simulink model "SF103A_MotRefMdl"  (R2013b)
settings: Solver=FixedStepDiscrete  StartTime=0.0  StopTime=2  FixedStep=.002  RelTol=1e-3
values from neighbouring files (symbols this model uses):
  ARCHGLBPRM_2MILLISEC_SEC_F32 = DataDict.Constant    [SF103A_MotRefMdl_DataDict.m]
  ARCHGLBPRM_2OVERSQRT3_ULS_F32 = DataDict.Constant    [SF103A_MotRefMdl_DataDict.m]
  ARCHGLBPRM_2PI_ULS_F32 = DataDict.Constant    [SF103A_MotRefMdl_DataDict.m]
  ARCHGLBPRM_4OVERSQRT3_ULS_F32 = DataDict.Constant    [SF103A_MotRefMdl_DataDict.m]
  ARCHGLBPRM_5PIOVER4_ULS_F32 = DataDict.Constant    [SF103A_MotRefMdl_DataDict.m]
  ARCHGLBPRM_FLOATZEROTHD_ULS_F32 = DataDict.Constant    [SF103A_MotRefMdl_DataDict.m]
  ARCHGLBPRM_HALFSQRT3_ULS_F32 = DataDict.Constant    [SF103A_MotRefMdl_DataDict.m]
  ARCHGLBPRM_PI_ULS_F32 = DataDict.Constant    [SF103A_MotRefMdl_DataDict.m]
  MotRefMdlCurrDaxBoostGain = DataDict.Calibration    [SF103A_MotRefMdl_DataDict.m]
  MotRefMdlCurrDaxQaxRefDelta = DataDict.Calibration    [SF103A_MotRefMdl_DataDict.m]
  MotRefMdlCurrItrnTolr = DataDict.Calibration    [SF103A_MotRefMdl_DataDict.m]
  MotRefMdlFbCtrlDi = DataDict.Calibration    [SF103A_MotRefMdl_DataDict.m]
  MotRefMdlIvtrDeadTiBrdgVltgSca = DataDict.Calibration    [SF103A_MotRefMdl_DataDict.m]
  MotRefMdlMinCurrItrnLim = DataDict.Calibration    [SF103A_MotRefMdl_DataDict.m]
  MotRefMdlMotCurrDaxMaxSca = DataDict.Calibration    [SF103A_MotRefMdl_DataDict.m]
  MotRefMdlMotVltgDerivtvTiCon = DataDict.Calibration    [SF103A_MotRefMdl_DataDict.m]
  MotRefMdlRefLocnItrnLim = DataDict.Calibration    [SF103A_MotRefMdl_DataDict.m]
  MotRefMdlTqItrnLim = DataDict.Calibration    [SF103A_MotRefMdl_DataDict.m]
  MotRefMdlTqItrnTolr = DataDict.Calibration    [SF103A_MotRefMdl_DataDict.m]
  MotRefMdlVltgModDynCmpEna = DataDict.Calibration    [SF103A_MotRefMdl_DataDict.m]
  MotRefMdlVltgOverRThdSca = DataDict.Calibration    [SF103A_MotRefMdl_DataDict.m]
  SysGlbPrmMotPoleCnt = DataDict.ImprtdCal    [SF103A_MotRefMdl_DataDict.m]
undefined symbols (not defined in the file or in its folder): MotQuad1
libraries: NxtrLim x19, simulink x4, LnrIntrpn x3, Fil x2, NxtrAbslt x2, FixdToFloat x2, FloatToFixd x2, NxtrMath x1
(part 1 of 7)
settings Model: Creator=lzz0tm  LastModifiedBy=RZ2YLP
settings DataIOCC: LimitDataPoints=off  SaveFormat=Structure  SignalLogging=off  DSMLogging=off
settings OptimizationCC: BlockReduction=off  InlineParams=on  ZeroExternalMemoryAtStartup=off  ZeroInternalMemoryAtStartup=off  OptimizeModelRefInitCode=on  LifeSpan=1
settings DebuggingCC: SignalInfNanChecking=error  SignalRangeChecking=warning  UnderspecifiedInitializationDetection=Simplified  SolverPrmCheckMsg=error  InheritedTsInSrcMsg=error  DiscreteInheritContinuousMsg=error  SingleTaskRateTransMsg=error  TasksWithSamePriorityMsg=error  SigSpecEnsureSampleTimeMsg=error  CheckMatrixSingularityMsg=error  IntegerOverflowMsg=error  ParameterUnderflowMsg=error  ParameterPrecisionLossMsg=error  ParameterTunabilityLossMsg=error  FixptConstUnderflowMsg=warning  FixptConstOverflowMsg=warning  VectorMatrixConversionMsg=error  SignalLabelMismatchMsg=error  UnconnectedInputMsg=error  UnconnectedOutputMsg=error  UnconnectedLineMsg=error  SFcnCompatibilityMsg=error  UniqueDataStoreMsg=warning  BusObjectLabelMismatch=error  RootOutportRequireBusObject=error  AssertControl=DisableAll  ModelReferenceIOMsg=error  ModelReferenceVersionMismatchMessage=warning  ModelReferenceIOMismatchMessage=error  ModelReferenceCSMismatchMessage=warning  ModelReferenceDataLoggingMessage=error  StateNameClashWarn=warning  StrictBusMsg=ErrorOnBusTreatedAsVector  NonBusSignalsTreatedAsBus=error  SFUnexpectedBacktrackingDiag=error  SFInvalidInputDataAccessInChartInitDiag=error  SFNoUnconditionalDefaultTransitionDiag=error  SFTransitionOutsideNaturalParentDiag=error  SFUnconditionalTransitionShadowingDiag=error  SFUndirectedBroadcastEventsDiag=error
settings ModelReferenceCC: ModelReferenceNumInstancesAllowed=Single
settings RTWCC: SystemTargetFile=autosar.tlc  GenCodeOnly=on  TemplateMakefile=ert_default_tmf  Description=AUTOSAR  GenerateReport=on  ProcessScript=autosar_make_rtw_hook  LaunchReport=on
settings CodeAppCC: GenerateComments=off  IgnoreCustomStorageClasses=off  CustomSymbolStrType=$N$R$M  CustomSymbolStrBlkIO=$N$M  SimulinkBlockComments=off
settings STFCustomTargetCC: ParMdlRefBuildCompliant=on  CompOptLevelCompliant=on  IncludeMdlTerminateFcn=off  CombineOutputUpdateFcns=on  SuppressErrorStatus=on  ERTFirstTimeCompliant=on  ERTCustomFileBanners=on  SupportNonFinite=off  SupportComplex=off  SupportContinuousTime=off  SupportNonInlinedSFcns=off  MATLABClassNameForMDSCustomization=Simulink.SoftwareTarget.ERTCustomization  AutosarCompliant=on  GRTInterface=off  SystemTargetFile=autosar.tlc
settings ERTTargetCC: CodeReplacementLibrary=ANSI_C  ConcurrentExecutionCompliant=off  IncludeMdlTerminateFcn=off  SuppressErrorStatus=on  SupportNonFinite=off  SupportComplex=off  ModelStepFunctionPrototypeControlCompliant=off  CPPClassGenCompliant=off  AutosarCompliant=on  InlinedParameterPlacement=NonHierarchical  ERTCustomFileTemplate=example_file_process.tlc  EnableUserReplacementTypes=on

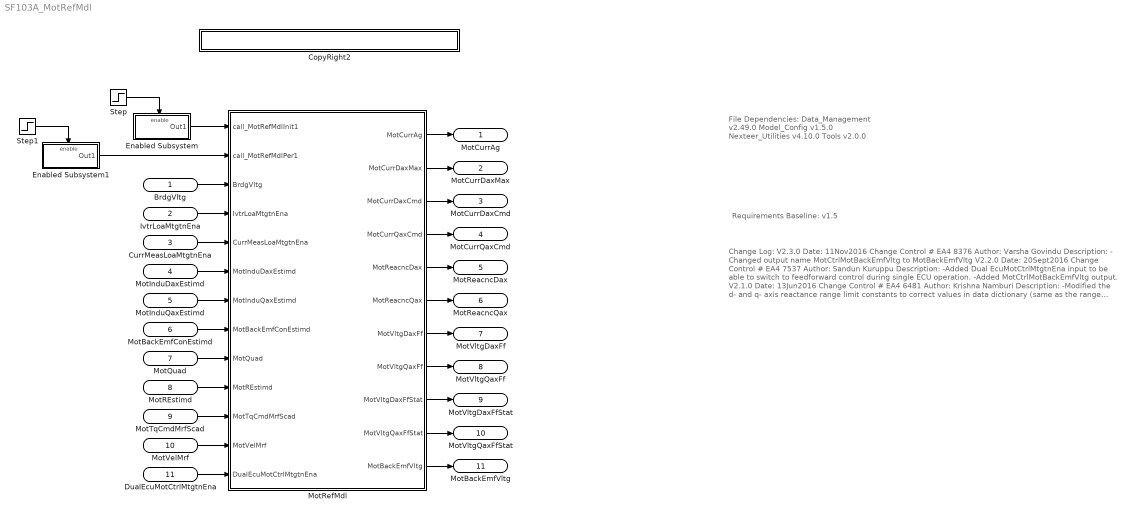
== system SF103A_MotRefMdl ==
  note: Requirements Baseline: v1.5
  note: File Dependencies:
      |
      | Data_Management v2.49.0
      | Model_Config v1.5.0
      | Nexteer_Utilities v4.10.0
      | Tools v2.0.0
  note: Change Log:
      |
      | V2.3.0
      | Date: 11Nov2016
      | Change Control # EA4 8376
      | Author: Varsha Govindu
      | Description:
      | - Changed  output name MotCtrlMotBackEmfVltg to MotBackEmfVltg
      |
      |
      | V2.2.0
      | Date: 20Sept2016
      | Change Control # EA4 7537
      | Author: Sandun Kuruppu
      | Description:
      | -Added Dual EcuMotCtrlMtgtnEna input to be able to switch to feedforward control during single
      | ECU operation.
      | -Added MotCtrlMotBackEmfVltg output.
      |
      | V2.1.0
      | Date: 13Jun2016
      | Change Control # EA4 6481
      | Author: Krishna Namburi
      | Description:
      | -Modified the d- and q- axis reactance range limit constants to correct values in data dictionary
      | (same as the range specified for the corresponding output signals).
      | -Corrected theDOORS requirement links for the output signals
      |
      | V2.0.0
      | Date: 13Jun2016
      | Change Control # EA46068
      | Author: Krishna Namburi
      | Description:
      | Added Saturation blocks to the feedforward voltage outputs.
      | Added two ouputs MotVltgDaxFfStat and MotVltgQaxFfStat
      |
      | V1.3.0
      | Date: 25Apr2016
      | Change Control: EA4#5437, EA4#5363, EA4#5505
      | DRW: Sudeep Shankar
      | Description:
      |
      | EA4#5437:
      | - Removed saturation block on the outputs MotVltgDaxFf and MotVltgQaxFf.
      | - Removed the constant  MOTVLTGLOLIM_VOLT_F32 from data dictionary as
      | it is no longer used.
      | - Changed the name of constant MOTVLTGHILIM_VOLT_F32 to
      | BRDGVLTGHILIM_VOLT_F32 in model and DD.
      | - Added saturation block on the inputs MotVelMrf and MotTqCmdMrfScad
      | - Added Motor velocity high and low limit constants and Motor Torque command
      | high and low limit constants in data dictionary.
      |
      | EA4#5363:
      | - Changed the name of the input signal 'MotCurrLoaMtgtnEna' to
      | 'CurrMeasLoaMtgtnEna' both in design and datadictionary
      |
      | EA4#5505:
      | - Added display variables for MotVltgDaxFfStat and MotVltgQaxFfStat
      |
      | V1.2.0
      | Date: 14Mar2016
      | Change Control: EA4#4665
      | DRW: Muragesh Asundi(KPIT)
      | Description:
      | Changed signal name from "MotCtrlMotCurrLoaMtgtnEna" to
      |  "MotCurrLoaMtgtnEna".
      |
      | V1.1.0
      | Date: 12Feb2016
      | Change Control: EA4#6578
      | DRW: Shailesh/Hemlata kamble/Muragesh(KPIT)
      | Description:
      | 1. Changed the inputs for calculation of "MotCurrDaxMax".
      | Used "MotInduDaxEstimd" instead of "MotInduQaxEstimd" as per EA4#2360
      | 2.Replaced "limiter block" with "if-else" logic as mentioned in EA4#2665
      | 3. Names of following have corrected as per AUTOSAR naming convention
      |
      | MotRefMdlCurrIterTol -> MotRefMdlCurrItrnTolr
      | MotRefMdlMinCurrIterLim -> MotRefMdlMinCurrItrnLim
      | MotRefMdlQ13VltgSdlX -> MotRefMdlQuad13VltgSdlX
      | MotRefMdlQ13VltgSdlY -> MotRefMdlQuad13VltgSdlY
      | MotRefMdlQ24VltgSdlX -> MotRefMdlQuad24VltgSdlX
      | MotRefMdlQ24VltgSdlY -> MotRefMdlQuad24VltgSdlY
      | MotRefMdlRefLocnIterLim -> MotRefMdlRefLocnItrnLim
      | MotRefMdlTqIterLim -> MotRefMdlTqItrnLim
      | MotRefMdlTqIterTol -> MotRefMdlTqItrnTolr
      | MotRefMdlVltgOvrRThdSca - MotRefMdlVltgOverRThdSca
      | dMotRefMdlPkTqNrItrn -> dMotRefMdlPeakTqNrItrn
      |
      | V1.0.0
      | Date: 19june2015
      | Change Control: EA4#285
      | DRW: Kevin Derry
      | Description:
      | - Initial Release
  BrdgVltg : Inport  RequirementInfo={} %GIDa_002e74ba_4d90_44d4_90c6_7a7ed3b84fe7
  IvtrLoaMtgtnEna : Inport  RequirementInfo={} %GIDa_a4fd61a5_cdd6_4e13_bb24_ad86140a0e25  Port=2
  CurrMeasLoaMtgtnEna : Inport  RequirementInfo={} %GIDa_c2a4c68b_2d87_4ecb_ac32_cc9aba368d56  Port=3
  MotInduDaxEstimd : Inport  RequirementInfo={} %GIDa_fe459d42_11f7_4520_8391_798b83d6a516  Port=4
  MotInduQaxEstimd : Inport  RequirementInfo={} %GIDa_0f6b35e5_2a2f_4a67_b96e_911dafdf4a7c  Port=5
  MotBackEmfConEstimd : Inport  RequirementInfo={} %GIDa_5b757b48_21e1_4bdd_bbe8_b25eaabed28d  Port=6
  MotQuad : Inport  RequirementInfo={} %GIDa_e10e4028_772a_461b_a96b_8e88bd788124  Port=7
  MotREstimd : Inport  RequirementInfo={} %GIDa_daff92ee_9fcb_4c1d_949c_c1b84c0d8058  Port=8
  MotTqCmdMrfScad : Inport  RequirementInfo={} %GIDa_5a505ccf_fd01_460a_b553_b9760a103946  Port=9
  MotVelMrf : Inport  RequirementInfo={} %GIDa_3a206742_0817_4b89_aaee_a915b460cff8  Port=10
  DualEcuMotCtrlMtgtnEna : Inport  RequirementInfo={} %GIDa_c709b502_2fd2_4013_acca_47a6e0722eaa  Port=11
  CopyRight2 : Subsystem  Description=|  mask(Copyright Information){none=on}
      | Copyright info block.                                               
      |                                                                     
      | Place copyright information at the top of every subsystem in design.
      mask prompts: none "No parameters"
      mask help: Place copyright information at the top of every subsystem in design.
      mask Display:
      | NxtrConf = 'Nexteer Confidential';
      | 
      | sys = bdroot; %handle for the current model ("system")
      | first = get_param(sys,'Created');
      | first = first(end-3:end);  %year is last four digits
      | 
      | last = get_param(sys,'LastModifiedDate');
      | if isempty(last)
      |     last = datestr(now,'yyyy');
      | else
      |     last = last(end-3:end);
      | end
      | 
      | if strcmp(first,last)
      |     fprintf('%s -- Copyright %s Nexteer',NxtrConf,first)
      | else
      |     fprintf('%s -- %s%s- %s Nexteer',NxtrConf,char(169),first,last)
      | end
  Enabled Subsystem : Subsystem  RequirementInfo={} %GIDa_5bd5b926_dcf2_442a_84c3_2b04d7299c9b  TreatAsAtomicUnit=on
  Enabled Subsystem1 : Subsystem  RequirementInfo={} %GIDa_aef5c3eb_1d89_4c7b_a89d_5c18a3b0f7b1  TreatAsAtomicUnit=on
  MotRefMdl : Subsystem  RequirementInfo={} %GIDa_b898030d_570f_4edd_8902_3dde318359c9
      settings: AttributesFormatString=%<Tag>
  Step : Step  RequirementInfo={} %GIDa_8c81d09d_84eb_4be8_baaa_75d0e6280a38  Time=.00001  Before=1  After=0  SampleTime=0.002
  Step1 : Step  RequirementInfo={} %GIDa_d7228de7_f622_4d51_9092_7c3999a0281d  Time=.00001  SampleTime=0.002
  MotCurrAg : Outport  RequirementInfo={} %GIDa_93cad014_54f9_4783_990f_6d2e5aad039b
  MotCurrDaxMax : Outport  RequirementInfo={} %GIDa_4136d505_73be_4586_8175_3cca54354780  Port=2
  MotCurrDaxCmd : Outport  RequirementInfo={} %GIDa_75f52d22_fe2b_494b_ac4f_7f4b1e1c25cf  Port=3
  MotCurrQaxCmd : Outport  RequirementInfo={} %GIDa_eb935c6c_ac14_4f59_8619_b2ab2e4003c8  Port=4
  MotReacncDax : Outport  RequirementInfo={} %GIDa_5d917e0d_38b8_4778_841b_e252e5a24515  Port=5
  MotReacncQax : Outport  RequirementInfo={} %GIDa_4b30cc88_72f0_4383_99ae_c006978f770d  Port=6
  MotVltgDaxFf : Outport  RequirementInfo={} %GIDa_44799714_324f_4cb8_bf73_cca9c6cf36e6  Port=7
  MotVltgQaxFf : Outport  RequirementInfo={} %GIDa_4412ce0c_324b_49e2_9e94_75936e15aac2  Port=8
  MotVltgDaxFfStat : Outport  RequirementInfo={} %GIDa_9d33dac4_1325_4267_bc65_d009f3dffb61  Port=9
  MotVltgQaxFfStat : Outport  RequirementInfo={} %GIDa_1d00fc51_e529_4e10_8bf6_e979105e5d3e  Port=10
  MotBackEmfVltg : Outport  RequirementInfo={} %GIDa_d7c5f473_23d1_4699_ab39_3d8c13b39e2e  Port=11
  wires:
  Enabled Subsystem1/1(Out1) -> MotRefMdl/2(call_MotRefMdlPer1)
  Enabled Subsystem/1(Out1) -> MotRefMdl/1(call_MotRefMdlInit1)
  Step/1 -> Enabled Subsystem/Enable
  MotRefMdl/6(MotReacncQax) -> MotReacncQax/1
  MotRefMdl/8(MotVltgQaxFf) -> MotVltgQaxFf/1
  MotRefMdl/7(MotVltgDaxFf) -> MotVltgDaxFf/1
  MotRefMdl/2(MotCurrDaxMax) -> MotCurrDaxMax/1
  MotRefMdl/4(MotCurrQaxCmd) -> MotCurrQaxCmd/1
  MotRefMdl/5(MotReacncDax) -> MotReacncDax/1
  MotRefMdl/3(MotCurrDaxCmd) -> MotCurrDaxCmd/1
  MotRefMdl/1(MotCurrAg) -> MotCurrAg/1
  CurrMeasLoaMtgtnEna/1 -> MotRefMdl/5(CurrMeasLoaMtgtnEna)
  MotInduQaxEstimd/1 -> MotRefMdl/7(MotInduQaxEstimd)
  IvtrLoaMtgtnEna/1 -> MotRefMdl/4(IvtrLoaMtgtnEna)
  MotInduDaxEstimd/1 -> MotRefMdl/6(MotInduDaxEstimd)
  MotBackEmfConEstimd/1 -> MotRefMdl/8(MotBackEmfConEstimd)
  BrdgVltg/1 -> MotRefMdl/3(BrdgVltg)
  MotQuad/1 -> MotRefMdl/9(MotQuad)
  MotREstimd/1 -> MotRefMdl/10(MotREstimd)
  MotVelMrf/1 -> MotRefMdl/12(MotVelMrf)
  MotTqCmdMrfScad/1 -> MotRefMdl/11(MotTqCmdMrfScad)
  MotRefMdl/10(MotVltgQaxFfStat) -> MotVltgQaxFfStat/1
  MotRefMdl/9(MotVltgDaxFfStat) -> MotVltgDaxFfStat/1
  MotRefMdl/11(MotBackEmfVltg) -> MotBackEmfVltg/1
  DualEcuMotCtrlMtgtnEna/1 -> MotRefMdl/13(DualEcuMotCtrlMtgtnEna)
  Step1/1 -> Enabled Subsystem1/Enable

== system SF103A_MotRefMdl/CopyRight2 ==

== system SF103A_MotRefMdl/Enabled Subsystem ==
  Enable : EnablePort
  Function-Call Generator : simulink/Ports & Subsystems/Function-Call Generator  sample_time=.002  numberOfIterations=1
  Out1 : Outport
  wires:
  Function-Call Generator/1 -> Out1/1

== system SF103A_MotRefMdl/Enabled Subsystem1 ==
  Enable : EnablePort
  Function-Call Generator : simulink/Ports & Subsystems/Function-Call Generator  sample_time=.002  numberOfIterations=1
  Out1 : Outport
  wires:
  Function-Call Generator/1 -> Out1/1

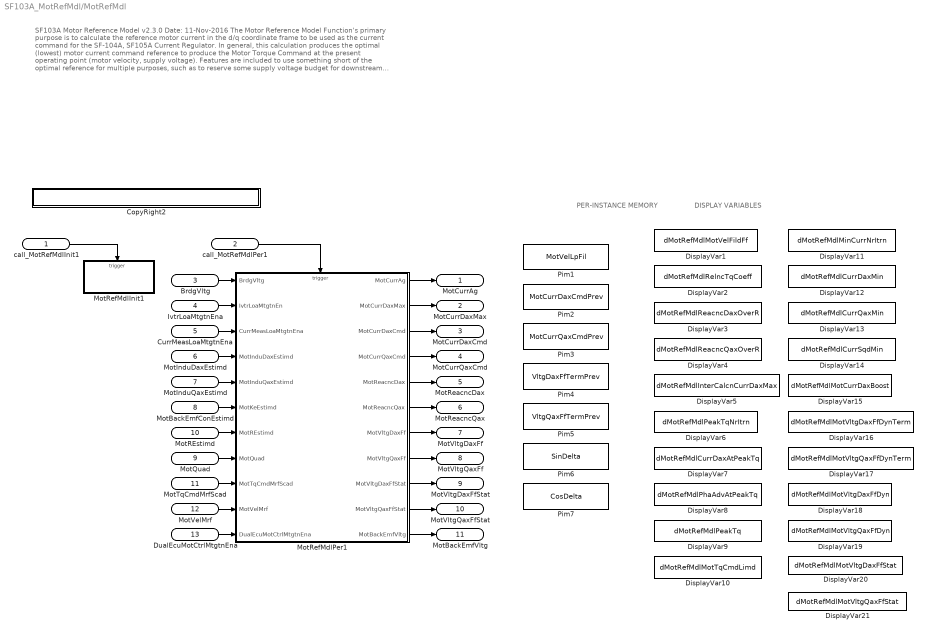
== system SF103A_MotRefMdl/MotRefMdl ==
  note: DISPLAY VARIABLES
  note: PER-INSTANCE
      | MEMORY
  note: SF103A  Motor Reference Model
      | v2.3.0      Date: 11-Nov-2016
      |
      | The Motor Reference Model Function's primary purpose is to calculate the reference motor current in the d/q coordinate frame to
      | be used as the current command for the SF-104A, SF105A Current Regulator.  In general, this calculation produces the optimal
      | (lowest) motor current command reference to produce the Motor Torque Command at the present operating point (motor velocity,
      |  supply voltage).  Features are included to use something short of the optimal reference for multiple purposes, such as to reserve
      |  some supply voltage budget for downstream current regulator operation, or for cogging/ripple cancellation, or to smooth the transition
      |  of low values of Id to high values of Id as the motor operating conditions change.  Supplementary functions include the calculation of a
      | Feedforward Reference Voltage for use in the SF-105A Current Regulator, whose form changes depending on the state of the signa
      | l LoA State (this allows operation in Voltage Mode Control in certain fail operational states).  Another supplementary function computes the
      |  Motor Reference Current angle (Alpha) for use in the Current Measurement function.
  call_MotRefMdlInit1 : Inport
  call_MotRefMdlPer1 : Inport  Port=2
  BrdgVltg : Inport  RequirementInfo={'linktype_rmi_doors' '0000bb42 (/E-STEER Core/SubSystem Specifications/Application Functions/SF99/SF103A Motor Reference Model)' '#SF103A_42' 'true' 'REQ:SF103A_42' '' } %GIDa_d3b1f893_8188_46d5_b395_9d7b6c4fbcc4  Port=3
  IvtrLoaMtgtnEna : Inport  RequirementInfo={'linktype_rmi_doors' '0000bb42 (/E-STEER Core/SubSystem Specifications/Application Functions/SF99/SF103A Motor Reference Model)' '#SF103A_183' 'true' 'REQ:SF103A_183' '' } %GIDa_c71961af_9957_4c72_9ff9_40a82d1c1450  Port=4
  CurrMeasLoaMtgtnEna : Inport  RequirementInfo={'linktype_rmi_doors' '0000bb42 (/E-STEER Core/SubSystem Specifications/Application Functions/SF99/SF103A Motor Reference Model)' '#SF103A_43' 'true' 'REQ:SF103A_43' '' } %GIDa_24854601_cc59_47b1_bc2c_d32f45ce8169  Port=5
  MotInduDaxEstimd : Inport  RequirementInfo={'linktype_rmi_doors' '0000bb42 (/E-STEER Core/SubSystem Specifications/Application Functions/SF99/SF103A Motor Reference Model)' '#SF103A_39' 'true' 'REQ:SF103A_39' '' } %GIDa_d84c7e48_30a1_4e89_aeaa_9b2784ab142a  Port=6
  MotInduQaxEstimd : Inport  RequirementInfo={'linktype_rmi_doors' '0000bb42 (/E-STEER Core/SubSystem Specifications/Application Functions/SF99/SF103A Motor Reference Model)' '#SF103A_40' 'true' 'REQ:SF103A_40' '' } %GIDa_2edb5c24_fcdf_496b_ab32_7ad89ca27fdb  Port=7
  MotBackEmfConEstimd : Inport  RequirementInfo={'linktype_rmi_doors' '0000bb42 (/E-STEER Core/SubSystem Specifications/Application Functions/SF99/SF103A Motor Reference Model)' '#SF103A_37' 'true' 'REQ:SF103A_37' '' } %GIDa_5a4a70dc_38a8_4966_aa75_58c98909303e  Port=8
  MotQuad : Inport  RequirementInfo={'linktype_rmi_doors' '0000bb42 (/E-STEER Core/SubSystem Specifications/Application Functions/SF99/SF103A Motor Reference Model)' '#SF103A_41' 'true' 'REQ:SF103A_41' '' } %GIDa_acb8662c_f7ec_4e47_adb3_a0fa4bbfd4b9  Port=9
  MotREstimd : Inport  RequirementInfo={'linktype_rmi_doors' '0000bb42 (/E-STEER Core/SubSystem Specifications/Application Functions/SF99/SF103A Motor Reference Model)' '#SF103A_38' 'true' 'REQ:SF103A_38' '' } %GIDa_d7c155ac_593d_4c0d_b2cd_a76dbcfddff9  Port=10
  MotTqCmdMrfScad : Inport  RequirementInfo={'linktype_rmi_doors' '0000bb42 (/E-STEER Core/SubSystem Specifications/Application Functions/SF99/SF103A Motor Reference Model)' '#SF103A_27' 'true' 'REQ:SF103A_27' '' } %GIDa_3d3c202a_f654_45d5_8a5b_acbb1c7e6aa0  Port=11
  MotVelMrf : Inport  RequirementInfo={'linktype_rmi_doors' '0000bb42 (/E-STEER Core/SubSystem Specifications/Application Functions/SF99/SF103A Motor Reference Model)' '#SF103A_36' 'true' 'REQ:SF103A_36' '' } %GIDa_7d8dfaf1_29d4_42ed_9984_abcaa0131fe4  Port=12
  DualEcuMotCtrlMtgtnEna : Inport  RequirementInfo={'linktype_rmi_doors' '0000bb42 (/E-STEER Core/SubSystem Specifications/Application Functions/SF99/SF103A Motor Reference Model)' '#SF103A_36' 'true' 'REQ:SF103A_36' '' } %GIDa_62cd6ed4_e69a_42ee_9441_e0d528756875  Port=13
  CopyRight2 : Subsystem  Description=|  mask(Copyright Information){none=on}
      | Copyright info block.                                               
      |                                                                     
      | Place copyright information at the top of every subsystem in design.
      mask prompts: none "No parameters"
      mask help: Place copyright information at the top of every subsystem in design.
      mask Display:
      | NxtrConf = 'Nexteer Confidential';
      | 
      | sys = bdroot; %handle for the current model ("system")
      | first = get_param(sys,'Created');
      | first = first(end-3:end);  %year is last four digits
      | 
      | last = get_param(sys,'LastModifiedDate');
      | if isempty(last)
      |     last = datestr(now,'yyyy');
      | else
      |     last = last(end-3:end);
      | end
      | 
      | if strcmp(first,last)
      |     fprintf('%s -- Copyright %s Nexteer',NxtrConf,first)
      | else
      |     fprintf('%s -- %s%s- %s Nexteer',NxtrConf,char(169),first,last)
      | end
  DisplayVar1 : DataStoreMemory  DataStoreName=dMotRefMdlMotVelFildFf  ReadBeforeWriteMsg=warning  WriteAfterWriteMsg=warning  WriteAfterReadMsg=warning  StateMustResolveToSignalObject=on
  DisplayVar10 : DataStoreMemory  DataStoreName=dMotRefMdlMotTqCmdLimd  ReadBeforeWriteMsg=warning  WriteAfterWriteMsg=warning  WriteAfterReadMsg=warning  StateMustResolveToSignalObject=on
  DisplayVar11 : DataStoreMemory  DataStoreName=dMotRefMdlMinCurrNrItrn  ReadBeforeWriteMsg=warning  WriteAfterWriteMsg=warning  WriteAfterReadMsg=warning  StateMustResolveToSignalObject=on
  DisplayVar12 : DataStoreMemory  DataStoreName=dMotRefMdlCurrDaxMin  ReadBeforeWriteMsg=warning  WriteAfterWriteMsg=warning  WriteAfterReadMsg=warning  StateMustResolveToSignalObject=on
  DisplayVar13 : DataStoreMemory  DataStoreName=dMotRefMdlCurrQaxMin  ReadBeforeWriteMsg=warning  WriteAfterWriteMsg=warning  WriteAfterReadMsg=warning  StateMustResolveToSignalObject=on
  DisplayVar14 : DataStoreMemory  DataStoreName=dMotRefMdlCurrSqdMin  ReadBeforeWriteMsg=warning  WriteAfterWriteMsg=warning  WriteAfterReadMsg=warning  StateMustResolveToSignalObject=on
  DisplayVar15 : DataStoreMemory  DataStoreName=dMotRefMdlMotCurrDaxBoost  ReadBeforeWriteMsg=warning  WriteAfterWriteMsg=warning  WriteAfterReadMsg=warning  StateMustResolveToSignalObject=on
  DisplayVar16 : DataStoreMemory  DataStoreName=dMotRefMdlMotVltgDaxFfDynTerm  ReadBeforeWriteMsg=warning  WriteAfterWriteMsg=warning  WriteAfterReadMsg=warning  StateMustResolveToSignalObject=on
  DisplayVar17 : DataStoreMemory  DataStoreName=dMotRefMdlMotVltgQaxFfDynTerm  ReadBeforeWriteMsg=warning  WriteAfterWriteMsg=warning  WriteAfterReadMsg=warning  StateMustResolveToSignalObject=on
  DisplayVar18 : DataStoreMemory  DataStoreName=dMotRefMdlMotVltgDaxFfDyn  ReadBeforeWriteMsg=warning  WriteAfterWriteMsg=warning  WriteAfterReadMsg=warning  StateMustResolveToSignalObject=on
  DisplayVar19 : DataStoreMemory  DataStoreName=dMotRefMdlMotVltgQaxFfDyn  ReadBeforeWriteMsg=warning  WriteAfterWriteMsg=warning  WriteAfterReadMsg=warning  StateMustResolveToSignalObject=on
  DisplayVar2 : DataStoreMemory  DataStoreName=dMotRefMdlRelncTqCoeff  ReadBeforeWriteMsg=warning  WriteAfterWriteMsg=warning  WriteAfterReadMsg=warning  StateMustResolveToSignalObject=on
  DisplayVar20 : DataStoreMemory  DataStoreName=dMotRefMdlMotVltgDaxFfStat  ReadBeforeWriteMsg=warning  WriteAfterWriteMsg=warning  WriteAfterReadMsg=warning  StateMustResolveToSignalObject=on
  DisplayVar21 : DataStoreMemory  DataStoreName=dMotRefMdlMotVltgQaxFfStat  ReadBeforeWriteMsg=warning  WriteAfterWriteMsg=warning  WriteAfterReadMsg=warning  StateMustResolveToSignalObject=on
  DisplayVar3 : DataStoreMemory  DataStoreName=dMotRefMdlReacncDaxOverR  ReadBeforeWriteMsg=warning  WriteAfterWriteMsg=warning  WriteAfterReadMsg=warning  StateMustResolveToSignalObject=on
  DisplayVar4 : DataStoreMemory  DataStoreName=dMotRefMdlReacncQaxOverR  ReadBeforeWriteMsg=warning  WriteAfterWriteMsg=warning  WriteAfterReadMsg=warning  StateMustResolveToSignalObject=on
  DisplayVar5 : DataStoreMemory  DataStoreName=dMotRefMdlInterCalcnCurrDaxMax  ReadBeforeWriteMsg=warning  WriteAfterWriteMsg=warning  WriteAfterReadMsg=warning  StateMustResolveToSignalObject=on
  DisplayVar6 : DataStoreMemory  DataStoreName=dMotRefMdlPeakTqNrItrn  ReadBeforeWriteMsg=warning  WriteAfterWriteMsg=warning  WriteAfterReadMsg=warning  StateMustResolveToSignalObject=on
  DisplayVar7 : DataStoreMemory  DataStoreName=dMotRefMdlCurrDaxAtPeakTq  ReadBeforeWriteMsg=warning  WriteAfterWriteMsg=warning  WriteAfterReadMsg=warning  StateMustResolveToSignalObject=on
  DisplayVar8 : DataStoreMemory  DataStoreName=dMotRefMdlPhaAdvAtPeakTq  ReadBeforeWriteMsg=warning  WriteAfterWriteMsg=warning  WriteAfterReadMsg=warning  StateMustResolveToSignalObject=on
  DisplayVar9 : DataStoreMemory  DataStoreName=dMotRefMdlPeakTq  ReadBeforeWriteMsg=warning  WriteAfterWriteMsg=warning  WriteAfterReadMsg=warning  StateMustResolveToSignalObject=on
  MotRefMdlInit1 : Subsystem  TreatAsAtomicUnit=on
  MotRefMdlPer1 : Subsystem  TreatAsAtomicUnit=on
  Pim1 : DataStoreMemory  DataStoreName=MotVelLpFil  InitialValue=struct('FilSt',single(0),'FilGain',single(0))  OutDataTypeStr=Bus: FilLpRec1  StateMustResolveToSignalObject=on
  Pim2 : DataStoreMemory  DataStoreName=MotCurrDaxCmdPrev  WriteAfterWriteMsg=warning  StateMustResolveToSignalObject=on
  Pim3 : DataStoreMemory  DataStoreName=MotCurrQaxCmdPrev  WriteAfterWriteMsg=warning  StateMustResolveToSignalObject=on
  Pim4 : DataStoreMemory  DataStoreName=VltgDaxFfTermPrev  WriteAfterWriteMsg=warning  StateMustResolveToSignalObject=on
  Pim5 : DataStoreMemory  DataStoreName=VltgQaxFfTermPrev  WriteAfterWriteMsg=warning  StateMustResolveToSignalObject=on
  Pim6 : DataStoreMemory  DataStoreName=SinDelta  WriteAfterWriteMsg=warning  InitialValue=[0 0 0 0 0 0 0 0]  StateMustResolveToSignalObject=on
  Pim7 : DataStoreMemory  DataStoreName=CosDelta  WriteAfterWriteMsg=warning  InitialValue=[0 0 0 0 0 0 0 0]  StateMustResolveToSignalObject=on
  MotCurrAg : Outport  RequirementInfo={'linktype_rmi_doors' '0000bb42 (/E-STEER Core/SubSystem Specifications/Application Functions/SF99/SF103A Motor Reference Model)' '#SF103A_28' 'true' 'REQ:SF103A_28' '' } %GIDa_834cbc2e_f18c_4f09_adae_97704fe7531a
  MotCurrDaxMax : Outport  RequirementInfo={'linktype_rmi_doors' '0000bb42 (/E-STEER Core/SubSystem Specifications/Application Functions/SF99/SF103A Motor Reference Model)' '#SF103A_50' 'true' 'REQ:SF103A_50' '' } %GIDa_0574a43c_0095_465e_bbc3_0acf9fa9b1b8  Port=2
  MotCurrDaxCmd : Outport  RequirementInfo={'linktype_rmi_doors' '0000bb42 (/E-STEER Core/SubSystem Specifications/Application Functions/SF99/SF103A Motor Reference Model)' '#SF103A_45' 'true' 'REQ:SF103A_45' '' } %GIDa_fb157a0c_9e0a_4510_ba81_91b763a1b3b4  Port=3
  MotCurrQaxCmd : Outport  RequirementInfo={'linktype_rmi_doors' '0000bb42 (/E-STEER Core/SubSystem Specifications/Application Functions/SF99/SF103A Motor Reference Model)' '#SF103A_44' 'true' 'REQ:SF103A_44' '' } %GIDa_ec3cc1cf_2433_46bf_a532_04cbfbe0ffa2  Port=4
  MotReacncDax : Outport  RequirementInfo={'linktype_rmi_doors' '0000bb42 (/E-STEER Core/SubSystem Specifications/Application Functions/SF99/SF103A Motor Reference Model)' '#SF103A_49' 'true' 'REQ:SF103A_49' '' } %GIDa_97e983dd_3b16_40dc_8e10_e6499980e643  Port=5
  MotReacncQax : Outport  RequirementInfo={'linktype_rmi_doors' '0000bb42 (/E-STEER Core/SubSystem Specifications/Application Functions/SF99/SF103A Motor Reference Model)' '#SF103A_48' 'true' 'REQ:SF103A_48' '' } %GIDa_ad59918e_bb5f_4124_9238_114ac982f978  Port=6
  MotVltgDaxFf : Outport  RequirementInfo={'linktype_rmi_doors' '0000bb42 (/E-STEER Core/SubSystem Specifications/Application Functions/SF99/SF103A Motor Reference Model)' '#SF103A_47' 'true' 'REQ:SF103A_47' '' } %GIDa_a89b73f7_0999_4306_87c4_354c6cee061c  Port=7
  MotVltgQaxFf : Outport  RequirementInfo={'linktype_rmi_doors' '0000bb42 (/E-STEER Core/SubSystem Specifications/Application Functions/SF99/SF103A Motor Reference Model)' '#SF103A_46' 'true' 'REQ:SF103A_46' '' } %GIDa_3b2f5587_35c7_4629_a038_bbfce1200d31  Port=8
  MotVltgDaxFfStat : Outport  RequirementInfo={'linktype_rmi_doors' '0000bb42 (/E-STEER Core/SubSystem Specifications/Application Functions/SF99/SF103A Motor Reference Model)' '#SF103A_185' 'true' 'REQ:SF103A_185' '' } %GIDa_966cb850_afba_44e3_801f_09c3cd3e5e21  Port=9
  MotVltgQaxFfStat : Outport  RequirementInfo={'linktype_rmi_doors' '0000bb42 (/E-STEER Core/SubSystem Specifications/Application Functions/SF99/SF103A Motor Reference Model)' '#SF103A_184' 'true' 'REQ:SF103A_184' '' } %GIDa_3c4d5d68_c8f7_4475_b626_248aa50b2e24  Port=10
  MotBackEmfVltg : Outport  RequirementInfo={'linktype_rmi_doors' '0000bb42 (/E-STEER Core/SubSystem Specifications/Application Functions/SF99/SF103A Motor Reference Model)' '#SF103A_187' 'true' 'REQ:SF103A_187' '' } %GIDa_de4675c2_9a6c_40d6_a388_66e44b7ee260  Port=11
  wires:
  call_MotRefMdlInit1/1 -> MotRefMdlInit1/Trigger
  call_MotRefMdlPer1/1 -> MotRefMdlPer1/Trigger
  MotInduDaxEstimd/1 -> MotRefMdlPer1/4(MotInduDaxEstimd)
  MotTqCmdMrfScad/1 -> MotRefMdlPer1/9(MotTqCmdMrfScad)
  MotInduQaxEstimd/1 -> MotRefMdlPer1/5(MotInduQaxEstimd)
  MotVelMrf/1 -> MotRefMdlPer1/10(MotVelMrf)
  MotQuad/1 -> MotRefMdlPer1/8(MotQuad)
  IvtrLoaMtgtnEna/1 -> MotRefMdlPer1/2(IvtrLoaMtgtnEn)
  CurrMeasLoaMtgtnEna/1 -> MotRefMdlPer1/3(CurrMeasLoaMtgtnEna)
  BrdgVltg/1 -> MotRefMdlPer1/1(BrdgVltg)
  MotBackEmfConEstimd/1 -> MotRefMdlPer1/6(MotKeEstimd)
  MotREstimd/1 -> MotRefMdlPer1/7(MotREstimd)
  MotRefMdlPer1/1(MotCurrAg) -> MotCurrAg/1
  MotRefMdlPer1/7(MotVltgDaxFf) -> MotVltgDaxFf/1
  MotRefMdlPer1/2(MotCurrDaxMax) -> MotCurrDaxMax/1
  MotRefMdlPer1/6(MotReacncQax) -> MotReacncQax/1
  MotRefMdlPer1/4(MotCurrQaxCmd) -> MotCurrQaxCmd/1
  MotRefMdlPer1/3(MotCurrDaxCmd) -> MotCurrDaxCmd/1
  MotRefMdlPer1/5(MotReacncDax) -> MotReacncDax/1
  MotRefMdlPer1/8(MotVltgQaxFf) -> MotVltgQaxFf/1
  MotRefMdlPer1/10(MotVltgQaxFfStat) -> MotVltgQaxFfStat/1
  MotRefMdlPer1/9(MotVltgDaxFfStat) -> MotVltgDaxFfStat/1
  MotRefMdlPer1/11(MotBackEmfVltg) -> MotBackEmfVltg/1
  DualEcuMotCtrlMtgtnEna/1 -> MotRefMdlPer1/11(DualEcuMotCtrlMtgtnEna)

== system SF103A_MotRefMdl/MotRefMdl/CopyRight2 ==

== system SF103A_MotRefMdl/MotRefMdl/MotRefMdlInit1 ==
  note: An array of phase advance interpolation points
  function : TriggerPort  TriggerType=function-call
  Constant2 : Constant  RequirementInfo={'linktype_rmi_doors' '0000bb42 (/E-STEER Core/SubSystem Specifications/Application Functions/SF99/SF103A Motor Reference Model)' '#SF103A_92' 'true' 'REQ:SF103A_92' '' } %GIDa_da78c45d_0dc3_4ce5_ba56_4e557b79ff02  Value=MotRefMdlCurrDaxQaxRefDelta
  CopyRight2 : Subsystem  Description=|  mask(Copyright Information){none=on}
      | Copyright info block.                                               
      |                                                                     
      | Place copyright information at the top of every subsystem in design.
      mask prompts: none "No parameters"
      mask help: Place copyright information at the top of every subsystem in design.
      mask Display:
      | NxtrConf = 'Nexteer Confidential';
      | 
      | sys = bdroot; %handle for the current model ("system")
      | first = get_param(sys,'Created');
      | first = first(end-3:end);  %year is last four digits
      | 
      | last = get_param(sys,'LastModifiedDate');
      | if isempty(last)
      |     last = datestr(now,'yyyy');
      | else
      |     last = last(end-3:end);
      | end
      | 
      | if strcmp(first,last)
      |     fprintf('%s -- Copyright %s Nexteer',NxtrConf,first)
      | else
      |     fprintf('%s -- %s%s- %s Nexteer',NxtrConf,char(169),first,last)
      | end
  CosDelta : DataStoreWrite  DataStoreName=CosDelta
  FilLpInit : Fil/FilLpInit  RequirementInfo={'linktype_rmi_doors' '0000bb42 (/E-STEER Core/SubSystem Specifications/Application Functions/SF99/SF103A Motor Reference Model)' '#SF103A_132' 'true' 'REQ:SF103A_132' '' } %GIDa_a8b99e42_23aa_467e_aeec_80c45b4357e7  Ic=0  Ts=ARCHGLBPRM_2MILLISEC_SEC_F32  Freq=MotRefMdlMotVelLpFilFrq  StVar=MotVelLpFil
  SinDelta : DataStoreWrite  DataStoreName=SinDelta
  Trigonometric Function : Trigonometry  RequirementInfo={'linktype_rmi_doors' '0000bb42 (/E-STEER Core/SubSystem Specifications/Application Functions/SF99/SF103A Motor Reference Model)' '#SF103A_92' 'true' 'REQ:SF103A_92' '' } %GIDa_9d61e243_4e46_4d4f_89b1_b878dd7a23ad
  Trigonometric Function1 : Trigonometry  RequirementInfo={'linktype_rmi_doors' '0000bb42 (/E-STEER Core/SubSystem Specifications/Application Functions/SF99/SF103A Motor Reference Model)' '#SF103A_92' 'true' 'REQ:SF103A_92' '' } %GIDa_8ef282f1_90e0_42b9_ae6e_708183d3f92b  Operator=cos
  wires:
  Trigonometric Function1/1 -> CosDelta/1
  Trigonometric Function/1 -> SinDelta/1
  Constant2/1 -> Trigonometric Function1/1, Trigonometric Function/1

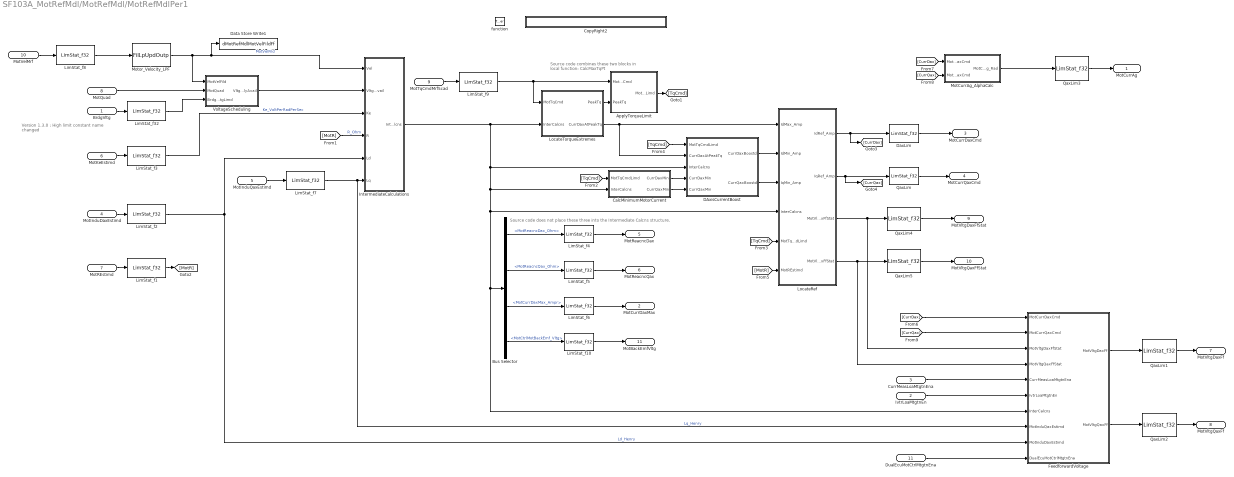
== system SF103A_MotRefMdl/MotRefMdl/MotRefMdlPer1 ==
  note: Version 1.3.0 : High limit constant name
      | changed
  note: Source code combines these two blocks
      | in local function: CalcMaxTqPt
  note: Source code does not place these three into the Intermediate Calcns structure.
  BrdgVltg : Inport
  IvtrLoaMtgtnEn : Inport  Port=2
  CurrMeasLoaMtgtnEna : Inport  Port=3
  MotInduDaxEstimd : Inport  Port=4
  MotInduQaxEstimd : Inport  Port=5
  MotKeEstimd : Inport  Port=6
  MotREstimd : Inport  Port=7
  MotQuad : Inport  Port=8
  MotTqCmdMrfScad : Inport  Port=9
  MotVelMrf : Inport  Port=10
  DualEcuMotCtrlMtgtnEna : Inport  RequirementInfo={'linktype_rmi_doors' '0000bb42 (/E-STEER Core/SubSystem Specifications/Application Functions/SF99/SF103A Motor Reference Model)' '#SF103A_36' 'true' 'REQ:SF103A_36' '' } %GIDa_e231b3f4_d483_40c0_9952_798d7510979a  Port=11
  function : TriggerPort  TriggerType=function-call
  ApplyTorqueLimit : Subsystem  RequirementInfo={'linktype_rmi_doors' '0000bb42 (/E-STEER Core/SubSystem Specifications/Application Functions/SF99/SF103A Motor Reference Model)' '#SF103A_177' 'true' 'REQ:SF103A_177' '' ; 'linktype_rmi_doors' '0000bb42 (/E-STEER Core/SubSystem Specifications/Application Functions/SF99/SF103A Motor Reference Model)' '#SF103A_102' 'true' 'REQ:SF103A_102' '' } %GIDa_4cf8c286_c687_497a_b145_e2429263c608
  Bus Selector : BusSelector  OutputSignals=MotReacncDax_Ohm,MotReacncQax_Ohm,MotCurrDaxMax_Ampr,MotCtrlMotBackEmf_Vltg
  CalcMinimumMotorCurrent : Subsystem  RequirementInfo={'linktype_rmi_doors' '0000bb42 (/E-STEER Core/SubSystem Specifications/Application Functions/SF99/SF103A Motor Reference Model)' '#SF103A_177' 'true' 'REQ:SF103A_177' '' } %GIDa_300b02b2_0762_4e99_94e0_c755190c5da5
  CopyRight2 : Subsystem  Description=|  mask(Copyright Information){none=on}
      | Copyright info block.                                               
      |                                                                     
      | Place copyright information at the top of every subsystem in design.
      mask prompts: none "No parameters"
      mask help: Place copyright information at the top of every subsystem in design.
      mask Display:
      | NxtrConf = 'Nexteer Confidential';
      | 
      | sys = bdroot; %handle for the current model ("system")
      | first = get_param(sys,'Created');
      | first = first(end-3:end);  %year is last four digits
      | 
      | last = get_param(sys,'LastModifiedDate');
      | if isempty(last)
      |     last = datestr(now,'yyyy');
      | else
      |     last = last(end-3:end);
      | end
      | 
      | if strcmp(first,last)
      |     fprintf('%s -- Copyright %s Nexteer',NxtrConf,first)
      | else
      |     fprintf('%s -- %s%s- %s Nexteer',NxtrConf,char(169),first,last)
      | end
  DAxisCurrentBoost : Subsystem  RequirementInfo={'linktype_rmi_doors' '0000bb42 (/E-STEER Core/SubSystem Specifications/Application Functions/SF99/SF103A Motor Reference Model)' '#SF103A_177' 'true' 'REQ:SF103A_177' '' } %GIDa_9c40fe5c_1486_43fb_8f9d_dcac451933b9
  Data Store Write1 : DataStoreWrite  DataStoreName=dMotRefMdlMotVelFildFf
  DaxLim : NxtrLim/LimStat_f32  RequirementInfo={'linktype_rmi_doors' '0000bb42 (/E-STEER Core/SubSystem Specifications/Application Functions/SF99/SF103A Motor Reference Model)' '#SF103A_68' 'true' 'REQ:SF103A_68' '' } %GIDa_516230ef_b2e3_4a6e_be94_d09f8f20f700  LoLim=0  HiLim=MOTCURRHILIM_AMPR_F32
      settings: AttributesFormatString=|
      | Low Limit: %<LoLim>
      | High Limit:%<HiLim>
  FeedforwardVoltage : Subsystem  RequirementInfo={'linktype_rmi_doors' '0000bb42 (/E-STEER Core/SubSystem Specifications/Application Functions/SF99/SF103A Motor Reference Model)' '#SF103A_177' 'true' 'REQ:SF103A_177' '' } %GIDa_b3e5d049_9911_4e4b_8475_2c7f4c9fe5fe
  IntermediateCalculations : Subsystem  RequirementInfo={'linktype_rmi_doors' '0000bb42 (/E-STEER Core/SubSystem Specifications/Application Functions/SF99/SF103A Motor Reference Model)' '#SF103A_177' 'true' 'REQ:SF103A_177' '' } %GIDa_7b3fdfc4_4104_4777_9b65_8135e4743913
  LimStat_f1 : NxtrLim/LimStat_f32  RequirementInfo={'linktype_rmi_doors' '0000bb42 (/E-STEER Core/SubSystem Specifications/Application Functions/SF99/SF103A Motor Reference Model)' '#SF103A_69' 'true' 'REQ:SF103A_69' '' } %GIDa_9b3a9daf_609e_49e6_8d22_3420d93cb324  LoLim=MOTRLOLIM_OHM_F32  HiLim=MOTRHILIM_OHM_F32
      settings: AttributesFormatString=|
      | Low Limit: %<LoLim>
      | High Limit:%<HiLim>
  LimStat_f10 : NxtrLim/LimStat_f32  RequirementInfo={'linktype_rmi_doors' '0000bb42 (/E-STEER Core/SubSystem Specifications/Application Functions/SF99/SF103A Motor Reference Model)' '#SF103A_188' 'true' 'REQ:SF103A_188' '' } %GIDa_bb6cd4c9_9324_4e39_95b7_18d9f501018b  LoLim=MOTBACKEMFVLTGLOLIM_VOLT_F32  HiLim=MOTBACKEMFVLTGHILIM_VOLT_F32
      settings: AttributesFormatString=|
      | Low Limit: %<LoLim>
      | High Limit:%<HiLim>
  LimStat_f2 : NxtrLim/LimStat_f32  RequirementInfo={'linktype_rmi_doors' '0000bb42 (/E-STEER Core/SubSystem Specifications/Application Functions/SF99/SF103A Motor Reference Model)' '#SF103A_69' 'true' 'REQ:SF103A_69' '' } %GIDa_d06208f0_c7d5_47ec_a449_88925d642ffb  LoLim=MOTINDULOLIM_HENRY_F32  HiLim=MOTINDUHILIM_HENRY_F32
      settings: AttributesFormatString=|
      | Low Limit: %<LoLim>
      | High Limit:%<HiLim>
  LimStat_f3 : NxtrLim/LimStat_f32  RequirementInfo={'linktype_rmi_doors' '0000bb42 (/E-STEER Core/SubSystem Specifications/Application Functions/SF99/SF103A Motor Reference Model)' '#SF103A_69' 'true' 'REQ:SF103A_69' '' } %GIDa_aa36a716_0843_4b34_8a71_b51a85e56c4a  LoLim=MOTBACKEMFCONLOLIM_VOLTPERMOTRADPERSEC_F32  HiLim=MOTBACKEMFCONHILIM_VOLTPERMOTRADPERSEC_F32
      settings: AttributesFormatString=|
      | Low Limit: %<LoLim>
      | High Limit:%<HiLim>
  LimStat_f32 : NxtrLim/LimStat_f32  RequirementInfo={'linktype_rmi_doors' '0000bb42 (/E-STEER Core/SubSystem Specifications/Application Functions/SF99/SF103A Motor Reference Model)' '#SF103A_69' 'true' 'REQ:SF103A_69' '' } %GIDa_8b94c28f_bf10_420e_8da1_14bdedfa1300  LoLim=BRDGVLTGLOLIM_VOLT_F32  HiLim=BRDGVLTGHILIM_VOLT_F32
      settings: AttributesFormatString=|
      | Low Limit: %<LoLim>
      | High Limit:%<HiLim>
  LimStat_f4 : NxtrLim/LimStat_f32  RequirementInfo={'linktype_rmi_doors' '0000bb42 (/E-STEER Core/SubSystem Specifications/Application Functions/SF99/SF103A Motor Reference Model)' '#SF103A_68' 'true' 'REQ:SF103A_68' '' } %GIDa_5afff691_2aa8_49d0_90d1_349ea980a360  LoLim=MOTREACNCLOLIM_OHM_F32  HiLim=MOTREACNCHILIM_OHM_F32
      settings: AttributesFormatString=|
      | Low Limit: %<LoLim>
      | High Limit:%<HiLim>
  LimStat_f5 : NxtrLim/LimStat_f32  RequirementInfo={'linktype_rmi_doors' '0000bb42 (/E-STEER Core/SubSystem Specifications/Application Functions/SF99/SF103A Motor Reference Model)' '#SF103A_68' 'true' 'REQ:SF103A_68' '' } %GIDa_92c3e442_84d7_4ab3_8ef1_1e782245d1e3  LoLim=MOTREACNCLOLIM_OHM_F32  HiLim=MOTREACNCHILIM_OHM_F32
      settings: AttributesFormatString=|
      | Low Limit: %<LoLim>
      | High Limit:%<HiLim>
  LimStat_f6 : NxtrLim/LimStat_f32  RequirementInfo={'linktype_rmi_doors' '0000bb42 (/E-STEER Core/SubSystem Specifications/Application Functions/SF99/SF103A Motor Reference Model)' '#SF103A_68' 'true' 'REQ:SF103A_68' '' } %GIDa_3b7b2b62_a855_4f8e_8ea4_9add98691729  LoLim=0  HiLim=MOTCURRHILIM_AMPR_F32
      settings: AttributesFormatString=|
      | Low Limit: %<LoLim>
      | High Limit:%<HiLim>
  LimStat_f7 : NxtrLim/LimStat_f32  RequirementInfo={'linktype_rmi_doors' '0000bb42 (/E-STEER Core/SubSystem Specifications/Application Functions/SF99/SF103A Motor Reference Model)' '#SF103A_69' 'true' 'REQ:SF103A_69' '' } %GIDa_b7cd772b_1f25_40c0_a694_81658663c9b2  LoLim=MOTINDULOLIM_HENRY_F32  HiLim=MOTINDUHILIM_HENRY_F32
      settings: AttributesFormatString=|
      | Low Limit: %<LoLim>
      | High Limit:%<HiLim>
  LimStat_f8 : NxtrLim/LimStat_f32  RequirementInfo={} %GIDa_e77a6e6d_78d2_4441_8ec4_a70a8e03138a  LoLim=MOTVELMRFLOLIM_MOTRADPERSEC_F32  HiLim=MOTVELMRFHILIM_MOTRADPERSEC_F32
      settings: AttributesFormatString=|
      | Low Limit: %<LoLim>
      | High Limit:%<HiLim>
  LimStat_f9 : NxtrLim/LimStat_f32  RequirementInfo={} %GIDa_e9bf250a_aee0_4e45_bd1d_b8933b460cb2  LoLim=SYSGLBPRM_MOTTQCMDLOLIM_MOTNWTMTR_F32  HiLim=SYSGLBPRM_MOTTQCMDHILIM_MOTNWTMTR_F32
      settings: AttributesFormatString=|
      | Low Limit: %<LoLim>
      | High Limit:%<HiLim>
  LocateRef : Subsystem  RequirementInfo={'linktype_rmi_doors' '0000bb42 (/E-STEER Core/SubSystem Specifications/Application Functions/SF99/SF103A Motor Reference Model)' '#SF103A_177' 'true' 'REQ:SF103A_177' '' } %GIDa_ddba18d1_c46f_47b7_9ac5_2682cb04bf11
  LocateTorqueExtremes : Subsystem  RequirementInfo={'linktype_rmi_doors' '0000bb42 (/E-STEER Core/SubSystem Specifications/Application Functions/SF99/SF103A Motor Reference Model)' '#SF103A_177' 'true' 'REQ:SF103A_177' '' } %GIDa_3044d871_1477_4081_83f9_79ca4a475aed
  MotCurrAg_AlphaCalc : Subsystem  RequirementInfo={'linktype_rmi_doors' '0000bb42 (/E-STEER Core/SubSystem Specifications/Application Functions/SF99/SF103A Motor Reference Model)' '#SF103A_177' 'true' 'REQ:SF103A_177' '' } %GIDa_b8c321e3_59ad_439e_abac_6bc7f5d721f0
  Motor_Velocity_LPF : Fil/FilLpUpdOutp  RequirementInfo={'linktype_rmi_doors' '0000bb42 (/E-STEER Core/SubSystem Specifications/Application Functions/SF99/SF103A Motor Reference Model)' '#SF103A_72' 'true' 'REQ:SF103A_72' '' } %GIDa_f1f5a218_80bb_454e_a449_f3eda6a21701  StVar=MotVelLpFil
      settings: AttributesFormatString=%<StVar>
  QaxLim : NxtrLim/LimStat_f32  RequirementInfo={'linktype_rmi_doors' '0000bb42 (/E-STEER Core/SubSystem Specifications/Application Functions/SF99/SF103A Motor Reference Model)' '#SF103A_68' 'true' 'REQ:SF103A_68' '' } %GIDa_7a3a22cb_e3f3_43b7_87b7_3eeb70d3b65a  LoLim=MOTCURRLOLIM_AMPR_F32  HiLim=MOTCURRHILIM_AMPR_F32
      settings: AttributesFormatString=|
      | Low Limit: %<LoLim>
      | High Limit:%<HiLim>
  QaxLim1 : NxtrLim/LimStat_f32  RequirementInfo={'linktype_rmi_doors' '0000bb42 (/E-STEER Core/SubSystem Specifications/Application Functions/SF99/SF103A Motor Reference Model)' '#SF103A_68' 'true' 'REQ:SF103A_68' '' } %GIDa_0df753b5_0b15_4097_9ea2_e0bd6b84ca82  LoLim=MOTVLTGDAXFFLOLIM_VOLT_F32  HiLim=MOTVLTGDAXFFHILIM_VOLT_F32
      settings: AttributesFormatString=|
      | Low Limit: %<LoLim>
      | High Limit:%<HiLim>
  QaxLim2 : NxtrLim/LimStat_f32  RequirementInfo={'linktype_rmi_doors' '0000bb42 (/E-STEER Core/SubSystem Specifications/Application Functions/SF99/SF103A Motor Reference Model)' '#SF103A_68' 'true' 'REQ:SF103A_68' '' } %GIDa_8116c8af_28d4_46ac_bffb_bee9780d103b  LoLim=MOTVLTGQAXFFLOLIM_VOLT_F32  HiLim=MOTVLTGQAXFFHILIM_VOLT_F32
      settings: AttributesFormatString=|
      | Low Limit: %<LoLim>
      | High Limit:%<HiLim>
  QaxLim3 : NxtrLim/LimStat_f32  RequirementInfo={'linktype_rmi_doors' '0000bb42 (/E-STEER Core/SubSystem Specifications/Application Functions/SF99/SF103A Motor Reference Model)' '#SF103A_68' 'true' 'REQ:SF103A_68' '' } %GIDa_e46fee5c_b412_4fde_925a_1395353c8f92  LoLim=0  HiLim=MOTCURRAGHILIM_MOTRAD_F32
      settings: AttributesFormatString=|
      | Low Limit: %<LoLim>
      | High Limit:%<HiLim>
  QaxLim4 : NxtrLim/LimStat_f32  RequirementInfo={'linktype_rmi_doors' '0000bb42 (/E-STEER Core/SubSystem Specifications/Application Functions/SF99/SF103A Motor Reference Model)' '#SF103A_68' 'true' 'REQ:SF103A_68' '' } %GIDa_c769ac10_8cfb_4527_b288_ca4564f0e081  LoLim=MOTVLTGSTATLOLIM_VOLT_F32  HiLim=MOTVLTGSTATHILIM_VOLT_F32
      settings: AttributesFormatString=|
      | Low Limit: %<LoLim>
      | High Limit:%<HiLim>
  QaxLim5 : NxtrLim/LimStat_f32  RequirementInfo={'linktype_rmi_doors' '0000bb42 (/E-STEER Core/SubSystem Specifications/Application Functions/SF99/SF103A Motor Reference Model)' '#SF103A_68' 'true' 'REQ:SF103A_68' '' } %GIDa_bc177ab5_c350_41ff_a1e2_6420442e70fe  LoLim=MOTVLTGSTATLOLIM_VOLT_F32  HiLim=MOTVLTGSTATHILIM_VOLT_F32
      settings: AttributesFormatString=|
      | Low Limit: %<LoLim>
      | High Limit:%<HiLim>
  VoltageScheduling : Subsystem  RequirementInfo={'linktype_rmi_doors' '0000bb42 (/E-STEER Core/SubSystem Specifications/Application Functions/SF99/SF103A Motor Reference Model)' '#SF103A_177' 'true' 'REQ:SF103A_177' '' } %GIDa_c6e9759b_d4af_4dcb_8df4_e95b15b64014
  MotCurrAg : Outport
  MotCurrDaxMax : Outport  Port=2
  MotCurrDaxCmd : Outport  Port=3
  MotCurrQaxCmd : Outport  Port=4
  MotReacncDax : Outport  Port=5
  MotReacncQax : Outport  Port=6
  MotVltgDaxFf : Outport  Port=7
  MotVltgQaxFf : Outport  Port=8
  MotVltgDaxFfStat : Outport  Port=9
  MotVltgQaxFfStat : Outport  Port=10
  MotBackEmfVltg : Outport  Port=11
  wires:
  BrdgVltg/1 -> LimStat_f32/1
  MotVelMrf/1 -> LimStat_f8/1
  LimStat_f32/1 -> VoltageScheduling/3(BrdgVltgLimd)
  MotQuad/1 -> VoltageScheduling/2(MotQuad)
  LimStat_f2/1 -> FeedforwardVoltage/9(MotInduDaxEstimd), IntermediateCalculations/5(Ld)  "Ld_Henry"
  LimStat_f7/1 -> IntermediateCalculations/6(Lq), FeedforwardVoltage/8(MotInduQaxEstimd)  "Lq_Henry"
  LimStat_f3/1 -> IntermediateCalculations/3(Ke)  "Ke_VoltPerRadPerSec"
  VoltageScheduling/1(VltgSplyAvail) -> IntermediateCalculations/2(VltgSplyAvail)
  ApplyTorqueLimit/1(MotTqCmdLimd) -> [TqCmd]
  LocateTorqueExtremes/1(PeakTq) -> ApplyTorqueLimit/2(PeakTq)
  IntermediateCalculations/1(InterCalcns) -> FeedforwardVoltage/7(InterCalcns), Bus Selector/1, LocateRef/4(InterCalcns), CalcMinimumMotorCurrent/2(InterCalcns), DAxisCurrentBoost/3(InterCalcns), LocateTorqueExtremes/2(InterCalcns)
  MotTqCmdMrfScad/1 -> LimStat_f9/1
  LocateTorqueExtremes/2(CurrDaxAtPeakTq) -> DAxisCurrentBoost/2(CurrDaxAtPeakTq), LocateRef/1(IdMax_Amp)
  CalcMinimumMotorCurrent/1(CurrDaxMin) -> DAxisCurrentBoost/4(CurrDaxMin)
  CalcMinimumMotorCurrent/2(CurrQaxMin) -> DAxisCurrentBoost/5(CurrQaxMin)
  DAxisCurrentBoost/1(CurrDaxBoostd) -> LocateRef/2(IdMin_Amp)
  DAxisCurrentBoost/2(CurrQaxBoostd) -> LocateRef/3(IqMin_Amp)
  [TqCmd] -> CalcMinimumMotorCurrent/1(MotTqCmdLimd)
  [TqCmd] -> LocateRef/5(MotTqCmdLimd)
  [TqCmd] -> DAxisCurrentBoost/1(MotTqCmdLimd)
  LocateRef/2(IqRef_Amp) -> [CurrQax], QaxLim/1
  LocateRef/1(IdRef_Amp) -> [CurrDax], DaxLim/1
  [MotR] -> IntermediateCalculations/4(R)  "R_Ohm"
  DaxLim/1 -> MotCurrDaxCmd/1
  MotCurrAg_AlphaCalc/1(MotCurrAg_Rad) -> QaxLim3/1
  Bus Selector/3 -> LimStat_f6/1  "<MotCurrDaxMax_Ampr>"
  Bus Selector/1 -> LimStat_f4/1  "<MotReacncDax_Ohm>"
  Bus Selector/2 -> LimStat_f5/1  "<MotReacncQax_Ohm>"
  IvtrLoaMtgtnEn/1 -> FeedforwardVoltage/6(IvtrLoaMtgtnEn)
  LocateRef/4(MotVltgQaxFfStat) -> FeedforwardVoltage/4(MotVltgQaxFfStat), QaxLim5/1
  CurrMeasLoaMtgtnEna/1 -> FeedforwardVoltage/5(CurrMeasLoaMtgtnEna)
  [MotR] -> LocateRef/6(MotREstimd)
  MotREstimd/1 -> LimStat_f1/1
  LimStat_f1/1 -> [MotR]
  MotInduDaxEstimd/1 -> LimStat_f2/1
  MotKeEstimd/1 -> LimStat_f3/1
  LimStat_f4/1 -> MotReacncDax/1
  LimStat_f5/1 -> MotReacncQax/1
  LimStat_f6/1 -> MotCurrDaxMax/1
  FeedforwardVoltage/1(MotVltgDaxFf) -> QaxLim1/1
  FeedforwardVoltage/2(MotVltgQaxFf) -> QaxLim2/1
  QaxLim3/1 -> MotCurrAg/1
  QaxLim/1 -> MotCurrQaxCmd/1
  [CurrDax] -> FeedforwardVoltage/1(MotCurrDaxCmd)
  [CurrDax] -> MotCurrAg_AlphaCalc/1(MotCurrDaxCmd)
  [CurrQax] -> MotCurrAg_AlphaCalc/2(MotCurrQaxCmd)
  [CurrQax] -> FeedforwardVoltage/2(MotCurrQaxCmd)
  Motor_Velocity_LPF/1 -> VoltageScheduling/1(MotVelFild), IntermediateCalculations/1(Vel), Data Store Write1/1  "MotVelFild"
  MotInduQaxEstimd/1 -> LimStat_f7/1
  LimStat_f8/1 -> Motor_Velocity_LPF/1
  LimStat_f9/1 -> LocateTorqueExtremes/1(MotTqCmd), ApplyTorqueLimit/1(MotTqCmd)
  QaxLim1/1 -> MotVltgDaxFf/1
  QaxLim2/1 -> MotVltgQaxFf/1
  LocateRef/3(MotVltgDaxFfStat) -> QaxLim4/1, FeedforwardVoltage/3(MotVltgDaxFfStat)
  QaxLim4/1 -> MotVltgDaxFfStat/1
  QaxLim5/1 -> MotVltgQaxFfStat/1
  DualEcuMotCtrlMtgtnEna/1 -> FeedforwardVoltage/10(DualEcuMotCtrlMtgtnEna)
  LimStat_f10/1 -> MotBackEmfVltg/1
  Bus Selector/4 -> LimStat_f10/1  "<MotCtrlMotBackEmf_Vltg>"

== system SF103A_MotRefMdl/MotRefMdl/MotRefMdlInit1/CopyRight2 ==

== system SF103A_MotRefMdl/MotRefMdl/MotRefMdlPer1/ApplyTorqueLimit ==
  note: pass-thru blocks
  MotTqCmd : Inport  RequirementInfo={} %GIDa_025c6779_9066_4c26_ac7c_c60ce040d302
  PeakTq : Inport  RequirementInfo={} %GIDa_b2cef569_5ac6_4023_b455_5bd3826089a9  Port=2
  Abs : Abs  RequirementInfo={'linktype_rmi_doors' '0000bb42 (/E-STEER Core/SubSystem Specifications/Application Functions/SF99/SF103A Motor Reference Model)' '#SF103A_102' 'true' 'REQ:SF103A_102' '' } %GIDa_0a8c4a31_5582_4ed5_a511_fc446f1c3802
  Abs1 : Abs  RequirementInfo={'linktype_rmi_doors' '0000bb42 (/E-STEER Core/SubSystem Specifications/Application Functions/SF99/SF103A Motor Reference Model)' '#SF103A_102' 'true' 'REQ:SF103A_102' '' } %GIDa_2b7d6e19_285c_4413_8db0_5b71cefe1f49
  CopyRight2 : Subsystem  Description=|  mask(Copyright Information){none=on}
      | Copyright info block.                                               
      |                                                                     
      | Place copyright information at the top of every subsystem in design.
      mask prompts: none "No parameters"
      mask help: Place copyright information at the top of every subsystem in design.
      mask Display:
      | NxtrConf = 'Nexteer Confidential';
      | 
      | sys = bdroot; %handle for the current model ("system")
      | first = get_param(sys,'Created');
      | first = first(end-3:end);  %year is last four digits
      | 
      | last = get_param(sys,'LastModifiedDate');
      | if isempty(last)
      |     last = datestr(now,'yyyy');
      | else
      |     last = last(end-3:end);
      | end
      | 
      | if strcmp(first,last)
      |     fprintf('%s -- Copyright %s Nexteer',NxtrConf,first)
      | else
      |     fprintf('%s -- %s%s- %s Nexteer',NxtrConf,char(169),first,last)
      | end
  DisplayVar : DataStoreWrite  DataStoreName=dMotRefMdlMotTqCmdLimd
  If : If  RequirementInfo={'linktype_rmi_doors' '0000bb42 (/E-STEER Core/SubSystem Specifications/Application Functions/SF99/SF103A Motor Reference Model)' '#SF103A_102' 'true' 'REQ:SF103A_102' '' } %GIDa_f89377aa_d854_4d40_a11f_6bbea04da2f3  NumInputs=2  IfExpression=u1 < u2
  If Action Subsystem : Subsystem  RequirementInfo={'linktype_rmi_doors' '0000bb42 (/E-STEER Core/SubSystem Specifications/Application Functions/SF99/SF103A Motor Reference Model)' '#SF103A_102' 'true' 'REQ:SF103A_102' '' } %GIDa_32770edd_4c45_4b2d_99de_6da2954c3238  TreatAsAtomicUnit=on
  If Action Subsystem1 : Subsystem  RequirementInfo={'linktype_rmi_doors' '0000bb42 (/E-STEER Core/SubSystem Specifications/Application Functions/SF99/SF103A Motor Reference Model)' '#SF103A_102' 'true' 'REQ:SF103A_102' '' } %GIDa_7552b223_197d_4ca3_8265_c39c5904183a  TreatAsAtomicUnit=on
  Merge : Merge  RequirementInfo={'linktype_rmi_doors' '0000bb42 (/E-STEER Core/SubSystem Specifications/Application Functions/SF99/SF103A Motor Reference Model)' '#SF103A_102' 'true' 'REQ:SF103A_102' '' } %GIDa_db886489_62db_4718_9827_489e9b249dd2
  MotTqCmdLimd : Outport  RequirementInfo={} %GIDa_be70fa3d_feb5_4f31_bfcb_09d432719c8e
  wires:
  MotTqCmd/1 -> If Action Subsystem/1(In1), Abs/1
  PeakTq/1 -> If Action Subsystem1/1(In1), Abs1/1
  Abs/1 -> If/1
  Abs1/1 -> If/2
  If/1 -> If Action Subsystem/Action
  If/2 -> If Action Subsystem1/Action
  If Action Subsystem/1(Out1) -> Merge/1
  If Action Subsystem1/1(Out1) -> Merge/2
  Merge/1 -> DisplayVar/1, MotTqCmdLimd/1
